simulink model "average_func"  (R2021a)
settings: Solver=FixedStepDiscrete  StartTime=0.0  StopTime=10.0  RelTol=1e-3  EnableMultiTasking=on
settings Model: Creator=elkny  LastModifiedBy=elkny
settings DataIOCC: ReturnWorkspaceOutputs=off
settings OptimizationCC: DefaultParameterBehavior=Inlined  InlineInvariantSignals=on  EnableMemcpy=off  LifeSpan=1  EfficientTunableParamExpr=on
settings DebuggingCC: UnderspecifiedInitializationDetection=Classic  MergeDetectMultiDrivingBlocksExec=none  SFMachineParentedDataDiag=warning  ArithmeticOperatorsInVariantConditions=warning
settings ModelReferenceCC: PropagateSignalLabelsOutOfModel=off
settings SFSimCC: MATLABDynamicMemAlloc=off  CustomCodeUndefinedFunction=UseInterfaceOnly
settings RTWCC: SystemTargetFile=ert.tlc  GenCodeOnly=on  TemplateMakefile=ert_default_tmf  GenerateReport=on  IncludeHyperlinkInReport=on  LaunchReport=on  GenerateTraceInfo=on  GenerateTraceReport=on  GenerateTraceReportSl=on  GenerateTraceReportSf=on  GenerateTraceReportEml=on
settings CodeAppCC: ForceParamTrailComments=on  IgnoreCustomStorageClasses=off  OperatorAnnotations=on  SimulinkDataObjDesc=on  SFDataObjDesc=on  MATLABFcnDesc=on  InsertBlockDesc=on  StateflowObjectComments=on  MATLABSourceComments=on
settings ERTTargetCC: MultiwordLength=2048  GenerateSampleERTMain=on  InlinedParameterPlacement=NonHierarchical  ERTCustomFileTemplate=example_file_process.tlc

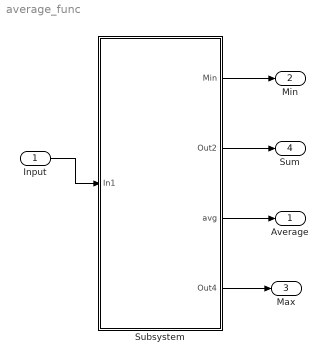
== system average_func ==
  Input : Inport
  Subsystem : Subsystem
  Average : Outport
  Min : Outport  Port=2
  Max : Outport  Port=3
  Sum : Outport  Port=4
  wires:
  Input/1 -> Subsystem/1(In1)
  Subsystem/2(Out2) -> Sum/1
  Subsystem/3(avg) -> Average/1
  Subsystem/4(Out4) -> Max/1
  Subsystem/1(Min) -> Min/1

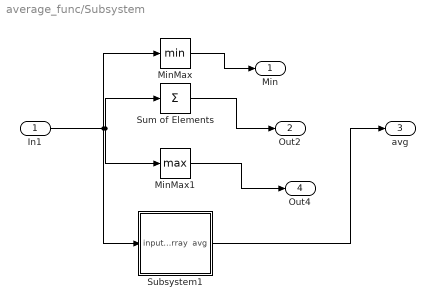
== system average_func/Subsystem ==
  In1 : Inport
  MinMax : MinMax
  MinMax1 : MinMax  Function=max
  Subsystem1 : Subsystem
  Sum of Elements : Sum  Inputs=+
  Min : Outport
  Out2 : Outport  Port=2
  avg : Outport  Port=3
  Out4 : Outport  Port=4
  wires:
  Sum of Elements/1 -> Out2/1
  MinMax/1 -> Min/1
  In1/1 -> Sum of Elements/1, MinMax1/1, MinMax/1, Subsystem1/1(inputArray)
  MinMax1/1 -> Out4/1
  Subsystem1/1(avg) -> avg/1

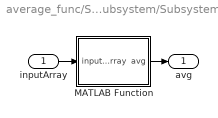
== system average_func/Subsystem/Subsystem1 ==
  inputArray : Inport
  MATLAB Function : MATLAB Function  TreatAsAtomicUnit=on
  avg : Outport
  wires:
  inputArray/1 -> MATLAB Function/1(inputArray)
  MATLAB Function/1(avg) -> avg/1

== matlab function average_func/Subsystem/Subsystem1/MATLAB Function ==
  data: inputArray input; avg output
function avg = calculateAverage(inputArray)
    avg = mean(inputArray);
end
